simulink model "simulink_client_hello_word"  (R2022b)
settings: Solver=FixedStepAuto  StartTime=0.0  StopTime=10.0  RelTol=1e-3
libraries: slrealtimeiplib x2, slrealtimeutilitieslib x1
settings Model: Creator=ramuj  LastModifiedBy=ramuj
settings SolverCC: ConcurrentTasks=on  PositivePriorityOrder=on
settings OptimizationCC: BlockReduction=off  OptimizeBlockIOStorage=off
settings DebuggingCC: TasksWithSamePriorityMsg=none
settings HardwareCC: ProdBitPerLong=64  ProdLongLongMode=on  ProdHWDeviceType=Intel->x86-64 (Linux 64)
settings RTWCC: Description=Simulink Real-Time  SystemTargetFile=slrealtime.tlc  TemplateMakefile=slrealtime_default_tmf  Toolchain=Simulink Real-Time Toolchain  BuildConfiguration=Faster Runs  CodeExecutionProfiling=on  TargetLang=C++

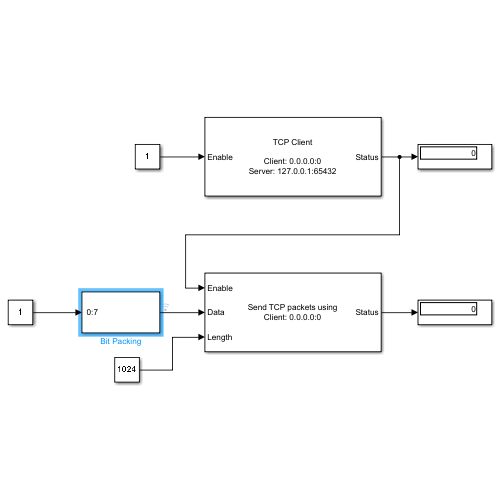
[thumbnail: Simulink's stored preview of the top-level diagram]
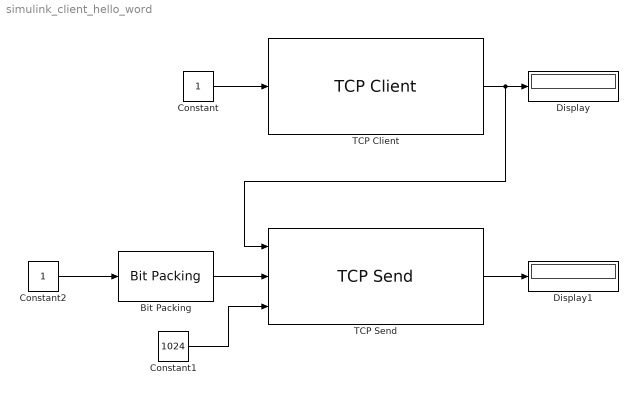
== system simulink_client_hello_word ==
  Bit Packing : slrealtimeutilitieslib/Bit Packing  MaskBitPatterns={[0:7]}  MaskPackDataType=uint8  MaskPackDataSize=[1024]
  Constant : Constant
  Constant1 : Constant  Value=1024
  Constant2 : Constant
  Display : Display
  Display1 : Display
  TCP Client : slrealtimeiplib/TCP Client  Priority=-1  useHostTargetConn=off  remoteAddress=HOST  remotePort=PORT
  TCP Send : slrealtimeiplib/TCP Send  socketAddPortVal=Client: 0.0.0.0:0  sampleTime=-1
  wires:
  Constant/1 -> TCP Client/1
  TCP Client/1 -> TCP Send/1, Display/1
  Constant2/1 -> Bit Packing/1
  TCP Send/1 -> Display1/1
  Constant1/1 -> TCP Send/3
  Bit Packing/1 -> TCP Send/2
